simulink model "MODEM_ASKbruit"  (R2020a)
settings: Solver=ode45  StartTime=0.0  StopTime=5000  RelTol=1e-3
libraries: commchan3 x1, commrandsrc2 x1, simulink x1, dsparch4 x1, commsink2 x1, dspsrcs4 x1, dspstat3 x1
settings Model: Creator=Administrateur  LastModifiedBy=J-MENTION
settings DataIOCC: LimitDataPoints=on  SaveFormat=Array  SignalLoggingSaveFormat=ModelDataLogs  ReturnWorkspaceOutputs=off
settings OptimizationCC: ExpressionDepthLimit=2147483647  InitFltsAndDblsToZero=on  LifeSpan=inf
settings DebuggingCC: UnderspecifiedInitializationDetection=Classic  MergeDetectMultiDrivingBlocksExec=none  SolverPrmCheckMsg=warning  FcnCallInpInsideContextMsg=warning  StateNameClashWarn=warning  SFUnexpectedBacktrackingDiag=warning  SFNoUnconditionalDefaultTransitionDiag=warning  SFExecutionAtInitializationDiag=none  ArithmeticOperatorsInVariantConditions=warning
settings HardwareCC: ProdBitPerPointer=32  ProdBitPerSizeT=32  ProdBitPerPtrDiffT=32  ProdLargestAtomicFloat=None  ProdIntDivRoundTo=Undefined  ProdEndianess=Unspecified  ProdWordSize=32  ProdHWDeviceType=32-bit Generic
settings ModelReferenceCC: PropagateSignalLabelsOutOfModel=off
settings SFSimCC: SimUseLocalCustomCode=off  CustomCodeUndefinedFunction=UseInterfaceOnly
settings RTWCC: RTWUseLocalCustomCode=off
settings CodeAppCC: StateflowObjectComments=on
settings GRTTargetCC: TargetLangStandard=C89/C90 (ANSI)  CombineOutputUpdateFcns=off  GRTInterface=on
settings ConfigComp: CovMetricSettings=dw  CovHtmlReporting=on  CovSaveCumulativeToWorkspaceVar=on  CovSaveSingleToWorkspaceVar=on  CovExternalEMLEnable=off

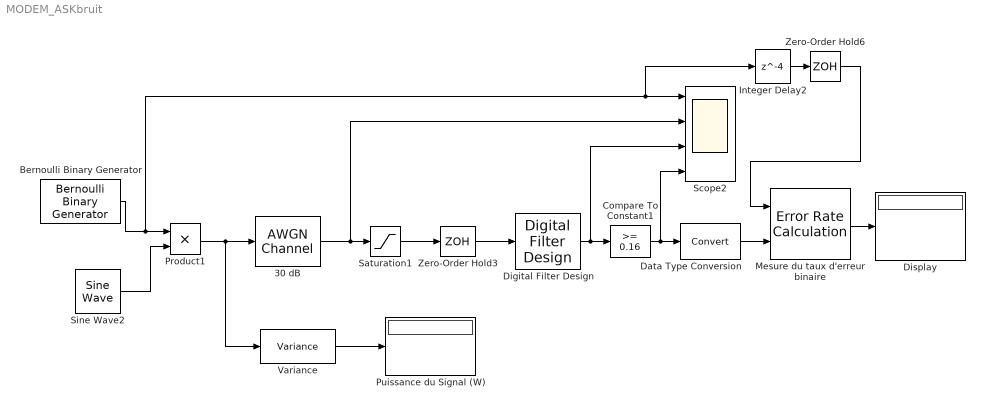
== system MODEM_ASKbruit ==
  30 dB : commchan3/AWGN Channel  InputProcessing=Columns as channels (frame based)  seed=67  noiseMode="Signal to noise ratio  (Eb/No)"  EbNodB=30  EsNodB=10  SNRdB=10  bitsPerSym=1  Ps=0.25  Tsym=1  variance=1
  Bernoulli Binary Generator : commrandsrc2/Bernoulli Binary Generator  P=0.5  seed=61  Ts=1  frameBased=off  sampPerFrame=1  orient=off  outDataType=double
      settings: SourceProductBaseCode=CM
  Compare To Constant1 : simulink/Logic and Bit Operations/Compare To Constant  relop=>=  const=0.16  OutDataTypeStr=uint8  ZeroCross=off
  Data Type Conversion : DataTypeConversion
  Digital Filter Design : dsparch4/Digital Filter Design  mwdsp_browser_bugfix_var=off
  Display : Display
  Integer Delay2 : Delay  DelayLength=4  SampleTime=1/100
  Mesure du taux d'erreur binaire : commsink2/Error Rate Calculation  N=0  st_delay=0  cp_mode=Entire frame  subframe=[]  PMode=Port  WsName=ErrorVec  RsMode2=off  stop=off  numErr=100  maxBits=1e6
  Product1 : Product  RndMeth=Zero
  Puissance du Signal (W) : Display
  Saturation1 : Saturate  UpperLimit=2  LowerLimit=0
  Scope2 : Scope  NumInputPorts=4
  Sine Wave2 : dspsrcs4/Sine Wave  Amplitude=1  Frequency=5  Phase=0  SampleMode=Discrete  OutComplex=Real  CompMethod=Trigonometric fcn  TableSize=Speed  SampleTime=1/100  SamplesPerFrame=1  ResetState=Restart at time zero  OutputFrames=on  dataType=double  wordLen=16  udDataType=sfix(16)  fracBitsMode=Best precision  numFracBits=15  OutDataTypeStr=double  LastOutDataTypeStr=double
  Variance : dspstat3/Variance  run=on  InputProcessing=Columns as channels (frame based)  reset_popup=None  directionMode=Each column  dimension=1  roiEnable=off  roiType=Rectangles  roiPortion=Entire ROI  roiOutput=Individual statistics for each ROI  roiFlag=off  roundingMode=Floor  overflowMode=off
  Zero-Order Hold3 : ZeroOrderHold  SampleTime=1e-2
  Zero-Order Hold6 : ZeroOrderHold
  wires:
  Bernoulli Binary Generator/1 -> Product1/1, Scope2/1, Integer Delay2/1
  Sine Wave2/1 -> Product1/2
  Mesure du taux d'erreur binaire/1 -> Display/1
  Digital Filter Design/1 -> Compare To Constant1/1, Scope2/3
  Compare To Constant1/1 -> Data Type Conversion/1, Scope2/4
  Product1/1 -> 30 dB/1, Variance/1
  30 dB/1 -> Scope2/2, Saturation1/1
  Saturation1/1 -> Zero-Order Hold3/1
  Zero-Order Hold3/1 -> Digital Filter Design/1
  Data Type Conversion/1 -> Mesure du taux d'erreur binaire/2
  Integer Delay2/1 -> Zero-Order Hold6/1
  Zero-Order Hold6/1 -> Mesure du taux d'erreur binaire/1
  Variance/1 -> Puissance du Signal (W)/1
